simulink model "simppend"  (R2018b)
settings: Solver=ode45  StartTime=0  StopTime=10  MaxStep=.1  RelTol=1e-3  AbsTol=1e-6
settings Model: ExtModeAutoUpdateStatusClock=off  Creator=The MathWorks, Inc.  LastModifiedBy=claudio.menghi
settings SolverCC: AutoScaleAbsTol=off
settings DataIOCC: ExternalInput=[]  InitialState=[]  SaveFormat=Array  SaveOutput=off  SaveTime=off
settings OptimizationCC: BlockReduction=off  BooleanDataType=off  InitFltsAndDblsToZero=on  LifeSpan=inf  BufferReusableBoundary=off
settings DebuggingCC: SaveWithParameterizedLinksMsg=none  SignalResolutionControl=TryResolveAllWithWarning  MultiTaskDSMMsg=warning  MultiTaskCondExecSysMsg=none  FcnCallInpInsideContextMsg=warning  BusObjectLabelMismatch=none  SFUnexpectedBacktrackingDiag=warning  SFNoUnconditionalDefaultTransitionDiag=warning  SFExecutionAtInitializationDiag=none
settings HardwareCC: ProdBitPerPointer=32  ProdBitPerSizeT=32  ProdBitPerPtrDiffT=32  ProdLargestAtomicFloat=None  ProdIntDivRoundTo=Undefined  ProdEndianess=Unspecified  ProdWordSize=32  ProdHWDeviceType=32-bit Generic  TargetUnknown=on
settings ModelReferenceCC: PropagateSignalLabelsOutOfModel=off
settings SFSimCC: SimUseLocalCustomCode=off
settings RTWCC: Description=Generic Real-Time Target  RTWUseLocalCustomCode=off
settings CodeAppCC: StateflowObjectComments=on
settings GRTTargetCC: TargetFcnLib=ansi_tfl_tmw.mat  TargetLangStandard=C89/C90 (ANSI)  GeneratePreprocessorConditionals=Disable all  CombineOutputUpdateFcns=off  GRTInterface=on
settings ConfigComp: CovMetricSettings=dw  CovHtmlReporting=on  CovSaveCumulativeToWorkspaceVar=on  CovSaveSingleToWorkspaceVar=on  CovExternalEMLEnable=off

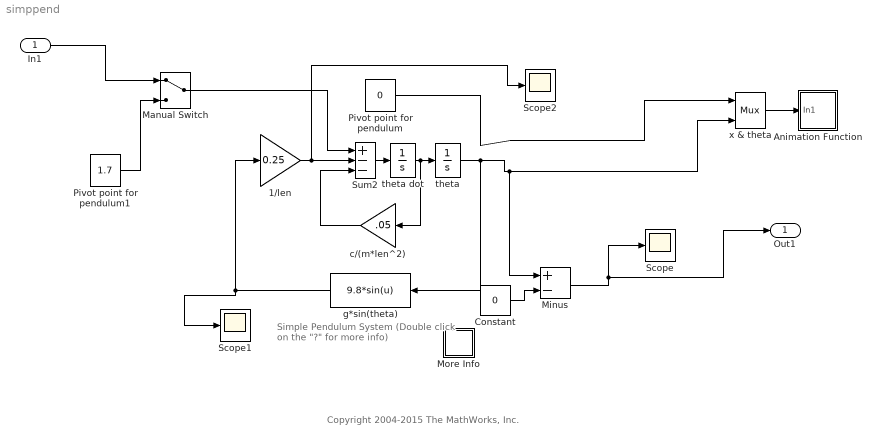
== system simppend ==
  note: Simple Pendulum System
      | (Double click on the "?" for more info)
  note: Copyright 2004-2015 The MathWorks, Inc.
  In1 : Inport
  1/len : Gain  Gain=0.25  SaturateOnIntegerOverflow=on  OutDataTypeStr=Inherit: Same as input  ParamDataTypeStr=Inherit: Same as input
  Animation Function : Subsystem  mask(Animation Block){ts=0.05}
      mask prompts: ts "Sample time:"
      mask Display: plot([.1,.9],[.9,.9],[.5,.2],[.9,.25],[.475,.475,.525,.525,.475],[.875,.925,.925,.875,.875])
  Constant : Constant  Value=0
  Manual Switch : ManualSwitch
  Minus : Sum  Inputs=+-
  More Info : Subsystem
      mask Display: disp('?')
  Pivot point for pendulum : Constant  Value=0
  Pivot point for pendulum1 : Constant  Value=1.7
  Scope : Scope
  Scope1 : Scope
  Scope2 : Scope
  Sum2 : Sum  Inputs=+--  SaturateOnIntegerOverflow=on  InputSameDT=on  OutDataTypeStr=Inherit: Same as first input
  c/(m*len^2) : Gain  Gain=.05  SaturateOnIntegerOverflow=on  OutDataTypeStr=Inherit: Same as input  ParamDataTypeStr=Inherit: Same as input
  g*sin(theta) : Fcn  Expr=9.8*sin(u)
  theta : Integrator  InitialCondition=1
  theta dot : Integrator
  x & theta : Mux  Inputs=2
  Out1 : Outport
  wires:
  Sum2/1 -> theta dot/1
  c/(m*len^2)/1 -> Sum2/3
  theta dot/1 -> c/(m*len^2)/1, theta/1
  Pivot point for pendulum/1 -> x & theta/1
  1/len/1 -> Scope2/1, Sum2/2
  g*sin(theta)/1 -> 1/len/1, Scope1/1
  x & theta/1 -> Animation Function/1(In1)
  Manual Switch/1 -> Sum2/1
  In1/1 -> Manual Switch/1
  theta/1 -> Minus/1, x & theta/2, g*sin(theta)/1
  Constant/1 -> Minus/2
  Minus/1 -> Out1/1, Scope/1
  Pivot point for pendulum1/1 -> Manual Switch/2

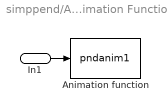
== system simppend/Animation Function ==
  In1 : Inport
  Animation function : S-Function  FunctionName=pndanim1  Parameters=ts  SFunctionDeploymentMode=off  EnableBusSupport=off
      settings: DeleteFcn=shh = get(0,'ShowHiddenHandles');set(0,'ShowHiddenHandles','on');if ~isempty(findobj('type','figure','name','simppend Animation'));close('simppend Animation'); end;set(0,'ShowHiddenHandles',shh);
  wires:
  In1/1 -> Animation function/1

== system simppend/More Info ==
  note: Associated with the example is an animation function that
      | will automatically open a figure window and display to it.
  note: This system models a simple pendulum system with
      | an applied external moment that varies periodically.
  note: Try experimenting with different initial conditions and
      | different setting for the applied moment M.
